simulink model "Simulink_MSDsystem-provided-by-the-instructor"  (R2023b)
settings: Solver=FixedStepAuto  StartTime=0.0  StopTime=3  FixedStep=0.02  RelTol=1e-3
settings Model: Creator=faraz.tehranizadeh  LastModifiedBy=faraz.tehranizadeh

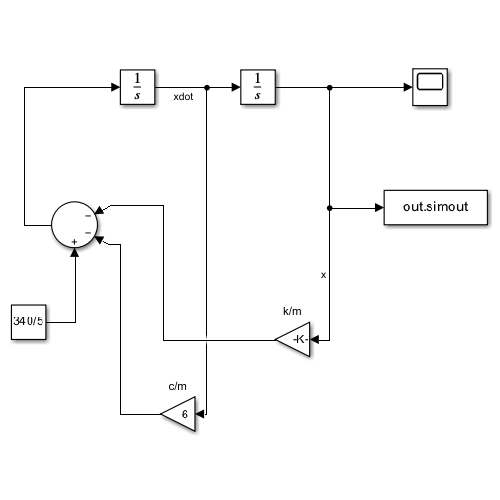
[thumbnail: Simulink's stored preview of the top-level diagram]
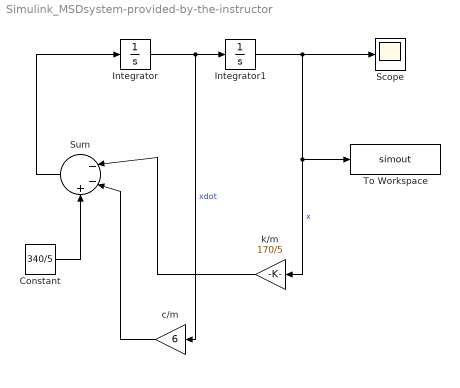
== system Simulink_MSDsystem-provided-by-the-instructor ==
  Constant : Constant  Value=340/5
  Integrator : Integrator
  Integrator1 : Integrator
  Scope : Scope
  Sum : Sum  Inputs=|--+
  To Workspace : ToWorkspace  VariableName=simout  SampleTime=-1
  c/m : Gain  Gain=6
  k/m : Gain  Gain=170/5
  wires:
  Integrator1/1 -> To Workspace/1, k/m/1, Scope/1  "x"
  Integrator/1 -> c/m/1, Integrator1/1  "xdot"
  Constant/1 -> Sum/3
  c/m/1 -> Sum/2
  k/m/1 -> Sum/1
  Sum/1 -> Integrator/1
